simulink subsystem "tehrani_tissue_mass_balance"  (R2019b)
settings: Solver=VariableStepAuto  StartTime=0.0  StopTime=10.0  RelTol=1e-3
settings Model: Creator=RH  LastModifiedBy=RH

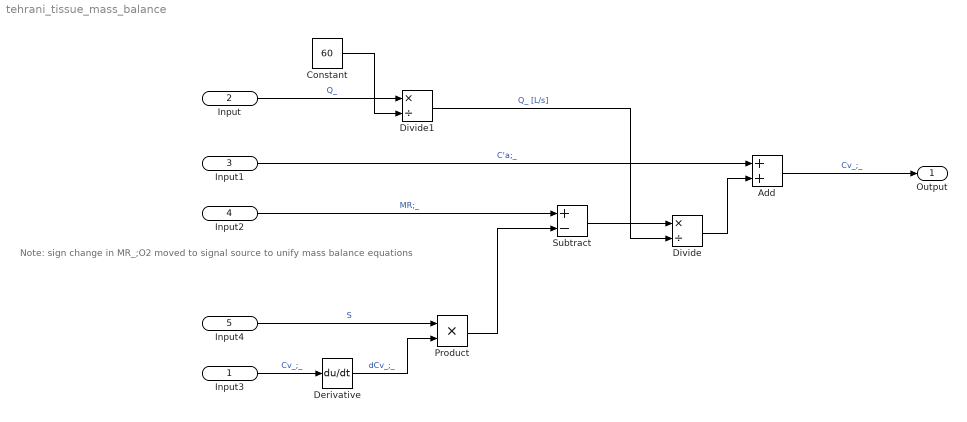
== system tehrani_tissue_mass_balance ==
  note: Note: sign change in MR_;O2 moved to signal source to unify mass balance equations
  Input3 : Inport  Unit=1
  Input : Inport  Port=2  Unit=liter/minute
  Input1 : Inport  Port=3  Unit=1
  Input2 : Inport  Port=4  Unit=liter/second
  Input4 : Inport  Port=5  Unit=liter
  Add : Sum
  Constant : Constant  Value=60
  Derivative : Derivative
  Divide : Product  Inputs=*/
  Divide1 : Product  Inputs=*/
  Product : Product
  Subtract : Sum  Inputs=+-
  Output : Outport  Unit=1
  wires:
  Divide1/1 -> Divide/2  "Q_ [L/s]"
  Derivative/1 -> Product/2  "dCv_;_"
  Add/1 -> Output/1  "Cv_;_"
  Product/1 -> Subtract/2
  Input4/1 -> Product/1  "S"
  Input3/1 -> Derivative/1  "Cv_;_"
  Divide/1 -> Add/2
  Subtract/1 -> Divide/1
  Input2/1 -> Subtract/1  "MR;_"
  Input1/1 -> Add/1  "C'a;_"
  Input/1 -> Divide1/1  "Q_"
  Constant/1 -> Divide1/2
